simulink model "main_RI_LIEKF_GNSSOutrage"  (R2023a)
settings: Solver=FixedStepAuto  StartTime=0.0  StopTime=220  FixedStep=0.01  RelTol=1e-3
InitFcn:
  | initNavigation0612_AOA;
values from neighbouring files (symbols this model uses):
  CF_enable = 0    [initNavigation.m]
  dt = 0.01    [initNavigation.m]
  dtDelay = -0.03    [initNavigation.m]
  g0 = 9.795    [initNavigation.m]
  gam0_rad = 0/57.3    (= 0)    [initNavigation.m]
  GNSSoutragetime = 90    [initNavigation.m]
  H_sensor_type = 0    [initNavigation.m]
  KF_enable = 1    [initNavigation.m]
  P0 = diag([1*ones(3,1);0.01*ones(3,1);0.1*ones(3,1);0.001*ones(3,1);0.00001*ones(3,1)])    [initNavigation.m]
  P0_RIEKF = diag([1*ones(3,1);0.01*ones(3,1);0.1*ones(3,1);0.001*ones(3,1);0.00001*ones(3,1);      0.01*ones(3,1);[0;2;2]/57.3;[0.1;0.1;0.1]])^2    [initNavigation.m]
  pd0 = 0    [initNavigation.m]
  pe0 = 0    [initNavigation.m]
  phi0_rad = 0/57.3    (= 0)    [initNavigation.m]
  pn0 = 0    [initNavigation.m]
  psi = -178    [initNavigation.m]
  psi0_rad = 0/57.3    (= 0)    [initNavigation.m]
  state_dim = 24    [initNavigation.m]
  Time = 0:0.01:(size(traindata.AttackAngle,1) - 1)*0.01    [NNLiftCoefficientFit.m]
  vd0 = 0    [initNavigation.m]
  ve0 = 0    [initNavigation.m]
  vn0 = 0    [initNavigation.m]
undefined symbols (not defined in the file or in its folder): DiscIntNeverNeededParam, Discrete, INS_CONST, INS_EXPORT, INS_PARAM, magnitude, p, param, pInitialization, sys
libraries: simulink_extras x94, simulink x82, dspstat3 x70, sharedtransform x60, ctrlSharedLib x36, sharedTrackingLibrary x22, matrix_library x15, FMT_Model_Lib x13, deeplib x8, dspsolvers x4, vrlib x4, aerolibconvert2 x1
(part 9 of 28)

== system main_RI_LIEKF_GNSSOutrage/State estimation/bak1/Error State Kalman Filter ==
  Sensor_data : Inport
  INS state : Inport  Port=2
  Add1 : Sum  Inputs=+-
  Add2 : Sum  Inputs=+-
  Bus Creator : BusCreator  Inputs=5
  Bus Selector : BusSelector  OutputSignals=QGC_sensor_reinit,GPS_Data.pos_N_gps,GPS_Data.pos_E_gps,GPS_Data.pos_D_gps,GPS_Data.vn_gps,GPS_Data.ve_gps,GPS_Data.vd_gps
  Bus Selector2 : BusSelector  OutputSignals=RotationData.DCM_b_n,INSstate_v,INSstste_p,INSstate_w,INSstate_fb
  Cal Q1 : Subsystem
  Constant1 : Constant  Value=diag([0.001,0.001,0.001,0.001,0.001,0.001])  OutDataTypeStr=single
  Data Store Read1 : DataStoreRead  DataStoreName=feedback_flag_18dim  IndexOptions=Index vector (dialog)  Indices=1  OutputSizes=1
  Data Store Read2 : DataStoreRead  DataStoreName=GPS_enable  IndexOptions=Index vector (dialog)  Indices=1  OutputSizes=1
  Data Store Read4 : DataStoreRead  DataStoreName=GPS_enable  IndexOptions=Index vector (dialog)  Indices=1  OutputSizes=1
  Data Store Read5 : DataStoreRead  DataStoreName=GPS_enable  IndexOptions=Index vector (dialog)  Indices=1  OutputSizes=1
  Data Store Read6 : DataStoreRead  DataStoreName=feedback_flag_18dim  IndexOptions=Index vector (dialog)  Indices=1  OutputSizes=1
  Data Store Write : DataStoreWrite  DataStoreName=GPS_enable  IndexOptions=Index vector (dialog)  Indices=1  OutputSizes=1
  Data Type Conversion{,1..2,6} (4 alike) : DataTypeConversion  OutDataTypeStr=single  SaturateOnIntegerOverflow=off  RndMeth=Floor
  Extended Kalman Filter1 : Subsystem  mask(Extended Kalman Filter){StateTransitionFcn=stateTransitionFcn_Dyn, HasStateTransitionJacobianFcn=off, StateTransitionJacobianFcn=stateTransitionJacobianFcn_Dyn, HasAdditiveProcessNoise=Nonadditive, ProcessNoise=1, HasTimeVaryingProcessNoise=on, HasStateTransitionFcnExtraArgument=0, InitialState=zeros(15,1), InitialStateCovariance=P0_RIEKF, MeasurementFcn1=GPSMeasurementFcn_Dyn, HasMeasurementJacobianFcn1=off, MeasurementJacobianFcn1=, HasMeasurementEnablePort1=on, HasAdditiveMeasurementNoise1=Nonadditive, MeasurementNoise1=1, HasTimeVaryingMeasurementNoise1=on, HasMeasurementFcnExtraArgument1=0, HasMeasurementWrapping1=off, MeasurementFcn2=ZUPTMeasurementFcn2, HasMeasurementJacobianFcn2=off, MeasurementJacobianFcn2=, HasMeasurementEnablePort2=on, HasAdditiveMeasurementNoise2=Nonadditive, MeasurementNoise2=1, HasTimeVaryingMeasurementNoise2=on, HasMeasurementFcnExtraArgument2=0, HasMeasurementWrapping2=off, MeasurementFcn3=ZUPTMeasurementFcn2, HasMeasurementJacobianFcn3=off, MeasurementJacobianFcn3=, HasMeasurementEnablePort3=on, HasAdditiveMeasurementNoise3=Nonadditive, MeasurementNoise3=1, HasTimeVaryingMeasurementNoise3=on, HasMeasurementFcnExtraArgument3=0, HasMeasurementWrapping3=off, MeasurementFcn4=myMeasurementFcn, HasMeasurementJacobianFcn4=off, MeasurementJacobianFcn4=, HasMeasurementEnablePort4=off, HasAdditiveMeasurementNoise4=Additive, MeasurementNoise4=1, HasTimeVaryingMeasurementNoise4=off, HasMeasurementFcnExtraArgument4=0, HasMeasurementWrapping4=off, MeasurementFcn5=myMeasurementFcn, HasMeasurementJacobianFcn5=off, MeasurementJacobianFcn5=, HasMeasurementEnablePort5=off, HasAdditiveMeasurementNoise5=Additive, MeasurementNoise5=1, HasTimeVaryingMeasurementNoise5=off, HasMeasurementFcnExtraArgument5=0, HasMeasurementWrapping5=off, EnableMultirate=off, StateTransitionFcnSampleTime=0.01, MeasurementFcn1SampleTime=0.2, MeasurementFcn2SampleTime=0.01, MeasurementFcn3SampleTime=1, MeasurementFcn4SampleTime=1, MeasurementFcn5SampleTime=1, UseCurrentEstimator=on, OutputStateCovariance=on, DataType=single, SampleTime=0.01, NumberOfMeasurements=1}
      mask prompts: HasStateTransitionJacobianFcn "shared_tracking:blocks:maskPromptEKFJacobian"; HasTimeVaryingProcessNoise "shared_tracking:blocks:maskPromptEKFUKFTimeVarying"; HasMeasurementJacobianFcn1 "shared_tracking:blocks:maskPromptEKFJacobian"; HasMeasurementEnablePort1 "shared_tracking:blocks:maskPromptEnablePort"; HasTimeVaryingMeasurementNoise1 "shared_tracking:blocks:maskPromptEKFUKFTimeVarying"; HasMeasurementWrapping1 "shared_tracking:blocks:maskPromptEKFUKFMeasurementWrapping"; HasMeasurementJacobianFcn2 "shared_tracking:blocks:maskPromptEKFJacobian"; HasMeasurementEnablePort2 "shared_tracking:blocks:maskPromptEnablePort"; HasTimeVaryingMeasurementNoise2 "shared_tracking:blocks:maskPromptEKFUKFTimeVarying"; HasMeasurementWrapping2 "shared_tracking:blocks:maskPromptEKFUKFMeasurementWrapping"; HasMeasurementJacobianFcn3 "shared_tracking:blocks:maskPromptEKFJacobian"; HasMeasurementEnablePort3 "shared_tracking:blocks:maskPromptEnablePort"; HasTimeVaryingMeasurementNoise3 "shared_tracking:blocks:maskPromptEKFUKFTimeVarying"; HasMeasurementWrapping3 "shared_tracking:blocks:maskPromptEKFUKFMeasurementWrapping"; HasMeasurementJacobianFcn4 "shared_tracking:blocks:maskPromptEKFJacobian"; HasMeasurementEnablePort4 "shared_tracking:blocks:maskPromptEnablePort"; HasTimeVaryingMeasurementNoise4 "shared_tracking:blocks:maskPromptEKFUKFTimeVarying"; HasMeasurementWrapping4 "shared_tracking:blocks:maskPromptEKFUKFMeasurementWrapping"; HasMeasurementJacobianFcn5 "shared_tracking:blocks:maskPromptEKFJacobian"; HasMeasurementEnablePort5 "shared_tracking:blocks:maskPromptEnablePort"; HasTimeVaryingMeasurementNoise5 "shared_tracking:blocks:maskPromptEKFUKFTimeVarying"; HasMeasurementWrapping5 "shared_tracking:blocks:maskPromptEKFUKFMeasurementWrapping"; EnableMultirate "shared_tracking:blocks:maskPromptEnableMultirate"; StateTransitionFcnSampleTime "shared_tracking:blocks:maskPromptStateTransition"; MeasurementFcn1SampleTime "shared_tracking:blocks:maskPromptMeasurement1"; MeasurementFcn2SampleTime "shared_tracking:blocks:maskPromptMeasurement2"; MeasurementFcn3SampleTime "shared_tracking:blocks:maskPromptMeasurement3"; MeasurementFcn4SampleTime "shared_tracking:blocks:maskPromptMeasurement4"; MeasurementFcn5SampleTime "shared_tracking:blocks:maskPromptMeasurement5"; UseCurrentEstimator "shared_tracking:blocks:maskPromptUseCurrentEstimator"; OutputStateCovariance "shared_tracking:blocks:maskPromptOutputStateCovariance"; DataType "shared_tracking:blocks:maskPromptDataType"; SampleTime "shared_tracking:blocks:maskPromptSampleTime"
      mask help: shared_tracking:blocks:maskPromptEKFDescription
      mask init:
      | matlabshared.tracking.internal.blocks.maskInitializationScriptEKF
      mask Help: eval('matlabshared.tracking.internal.blocks.controlIdentLaunchDocPage(''EKF'')')
      mask Callback HasStateTransitionJacobianFcn: matlabshared.tracking.internal.blocks.dialogCallbacksEKFUKFPF(gcbh(),'checkBoxHasJacobianFcn','StateTransition');
      mask TypeOptions HasAdditiveProcessNoise: shared_tracking:blocks:maskPromptEKFUKFAdditiveNoise | shared_tracking:blocks:maskPromptEKFUKFNonAdditiveNoise
      mask Callback HasTimeVaryingProcessNoise: matlabshared.tracking.internal.blocks.dialogCallbacksEKFUKFPF(gcbh,'checkboxIsCovarianceTimeVarying','HasTimeVaryingProcessNoise','ProcessNoise')
      mask Callback HasMeasurementJacobianFcn1: matlabshared.tracking.internal.blocks.dialogCallbacksEKFUKFPF(gcbh(),'checkBoxHasJacobianFcn','Measurement','1');
      mask TypeOptions HasAdditiveMeasurementNoise1: shared_tracking:blocks:maskPromptEKFUKFAdditiveNoise | shared_tracking:blocks:maskPromptEKFUKFNonAdditiveNoise
      mask Callback HasTimeVaryingMeasurementNoise1: matlabshared.tracking.internal.blocks.dialogCallbacksEKFUKFPF(gcbh,'checkboxIsCovarianceTimeVarying','HasTimeVaryingMeasurementNoise1','MeasurementNoise1')
      mask Callback HasMeasurementJacobianFcn2: matlabshared.tracking.internal.blocks.dialogCallbacksEKFUKFPF(gcbh(),'checkBoxHasJacobianFcn','Measurement','2');
      mask TypeOptions HasAdditiveMeasurementNoise2: shared_tracking:blocks:maskPromptEKFUKFAdditiveNoise | shared_tracking:blocks:maskPromptEKFUKFNonAdditiveNoise
      mask Callback HasTimeVaryingMeasurementNoise2: matlabshared.tracking.internal.blocks.dialogCallbacksEKFUKFPF(gcbh,'checkboxIsCovarianceTimeVarying','HasTimeVaryingMeasurementNoise2','MeasurementNoise2')
      mask Callback HasMeasurementJacobianFcn3: matlabshared.tracking.internal.blocks.dialogCallbacksEKFUKFPF(gcbh(),'checkBoxHasJacobianFcn','Measurement','3');
      mask TypeOptions HasAdditiveMeasurementNoise3: shared_tracking:blocks:maskPromptEKFUKFAdditiveNoise | shared_tracking:blocks:maskPromptEKFUKFNonAdditiveNoise
      mask Callback HasTimeVaryingMeasurementNoise3: matlabshared.tracking.internal.blocks.dialogCallbacksEKFUKFPF(gcbh,'checkboxIsCovarianceTimeVarying','HasTimeVaryingMeasurementNoise3','MeasurementNoise3')
      mask Callback HasMeasurementJacobianFcn4: matlabshared.tracking.internal.blocks.dialogCallbacksEKFUKFPF(gcbh(),'checkBoxHasJacobianFcn','Measurement','4');
      mask TypeOptions HasAdditiveMeasurementNoise4: shared_tracking:blocks:maskPromptEKFUKFAdditiveNoise | shared_tracking:blocks:maskPromptEKFUKFNonAdditiveNoise
      mask Callback HasTimeVaryingMeasurementNoise4: matlabshared.tracking.internal.blocks.dialogCallbacksEKFUKFPF(gcbh,'checkboxIsCovarianceTimeVarying','HasTimeVaryingMeasurementNoise4','MeasurementNoise4')
      mask Callback HasMeasurementJacobianFcn5: matlabshared.tracking.internal.blocks.dialogCallbacksEKFUKFPF(gcbh(),'checkBoxHasJacobianFcn','Measurement','5');
      mask TypeOptions HasAdditiveMeasurementNoise5: shared_tracking:blocks:maskPromptEKFUKFAdditiveNoise | shared_tracking:blocks:maskPromptEKFUKFNonAdditiveNoise
      mask Callback HasTimeVaryingMeasurementNoise5: matlabshared.tracking.internal.blocks.dialogCallbacksEKFUKFPF(gcbh,'checkboxIsCovarianceTimeVarying','HasTimeVaryingMeasurementNoise5','MeasurementNoise5')
      mask Callback EnableMultirate: matlabshared.tracking.internal.blocks.dialogCallbacksEKFUKFPF(gcbh,'checkBoxHasMultirate')
      mask TypeOptions DataType: shared_tracking:blocks:maskPromptDouble | shared_tracking:blocks:maskPromptSingle
      mask Callback NumberOfMeasurements: matlabshared.tracking.internal.blocks.dialogCallbacksEKFUKFPF(gcbh,'editboxNumberOfMeasurements','MeasurementFcn');
      mask DialogControl DescGroupVar Prompt: shared_tracking:blocks:maskPromptEKFTitle
      mask DialogControl TabSystemModel Prompt: shared_tracking:blocks:maskPromptSystemModel
      mask DialogControl GroupStateTransition Prompt: shared_tracking:blocks:maskPromptStateTransition
      mask DialogControl StateTransitionFunctionText Prompt: shared_tracking:blocks:maskPromptFunction
      mask DialogControl HasStateTransitionJacobianFcn Prompt: Jacobian
      mask DialogControl ProcessNoiseText Prompt: shared_tracking:blocks:maskPromptEKFUKFProcessNoise
      mask DialogControl ProcessNoiseCovarianceText Prompt: shared_tracking:blocks:maskPromptCovariance
      mask DialogControl HasTimeVaryingProcessNoise Prompt: Time-varying
      mask DialogControl InitializationContainer Prompt: shared_tracking:blocks:maskPromptInitialization
      mask DialogControl InitialStateText Prompt: shared_tracking:blocks:maskPromptEKFUKFInitialState
      mask DialogControl InitialCovarianceText Prompt: shared_tracking:blocks:maskPromptEKFUKFInitialCovariance
      mask DialogControl GroupMeasurement1 Prompt: shared_tracking:blocks:maskPromptMeasurement1
      mask DialogControl MeasurementFunction1Text Prompt: shared_tracking:blocks:maskPromptFunction
      mask DialogControl HasMeasurementJacobianFcn1 Prompt: Jacobian
      mask DialogControl HasMeasurementEnablePort1 Prompt: Add Enable port
      mask DialogControl MeasurementNoiseText1 Prompt: shared_tracking:blocks:maskPromptEKFUKFMeasurementNoise
      mask DialogControl MeasurementNoiseCovarianceText1 Prompt: shared_tracking:blocks:maskPromptCovariance
      mask DialogControl HasTimeVaryingMeasurementNoise1 Prompt: Time-varying
      mask DialogControl HasMeasurementWrapping1 Prompt: Has measurement wrapping
      mask DialogControl GroupMeasurement2 Prompt: shared_tracking:blocks:maskPromptMeasurement2
      mask DialogControl MeasurementFunction2Text Prompt: shared_tracking:blocks:maskPromptFunction
      mask DialogControl HasMeasurementJacobianFcn2 Prompt: Jacobian
      mask DialogControl HasMeasurementEnablePort2 Prompt: Add Enable port
      mask DialogControl MeasurementNoiseText2 Prompt: shared_tracking:blocks:maskPromptEKFUKFMeasurementNoise
      mask DialogControl MeasurementNoiseCovarianceText2 Prompt: shared_tracking:blocks:maskPromptCovariance
      mask DialogControl HasTimeVaryingMeasurementNoise2 Prompt: Time-varying
      mask DialogControl HasMeasurementWrapping2 Prompt: Has measurement wrapping
      mask DialogControl GroupMeasurement3 Prompt: shared_tracking:blocks:maskPromptMeasurement3
      mask DialogControl MeasurementFunction3Text Prompt: shared_tracking:blocks:maskPromptFunction
      mask DialogControl HasMeasurementJacobianFcn3 Prompt: Jacobian
      mask DialogControl HasMeasurementEnablePort3 Prompt: Add Enable port
      mask DialogControl MeasurementNoiseText3 Prompt: shared_tracking:blocks:maskPromptEKFUKFMeasurementNoise
      mask DialogControl MeasurementNoiseCovarianceText3 Prompt: shared_tracking:blocks:maskPromptCovariance
      mask DialogControl HasTimeVaryingMeasurementNoise3 Prompt: Time-varying
      mask DialogControl HasMeasurementWrapping3 Prompt: Has measurement wrapping
      mask DialogControl GroupMeasurement4 Prompt: shared_tracking:blocks:maskPromptMeasurement4
      mask DialogControl MeasurementFunction4Text Prompt: shared_tracking:blocks:maskPromptFunction
      mask DialogControl HasMeasurementJacobianFcn4 Prompt: Jacobian
      mask DialogControl HasMeasurementEnablePort4 Prompt: Add Enable port
      mask DialogControl MeasurementNoiseText4 Prompt: shared_tracking:blocks:maskPromptEKFUKFMeasurementNoise
      mask DialogControl MeasurementNoiseCovarianceText4 Prompt: shared_tracking:blocks:maskPromptCovariance
      mask DialogControl HasTimeVaryingMeasurementNoise4 Prompt: Time-varying
      mask DialogControl HasMeasurementWrapping4 Prompt: Has measurement wrapping
      mask DialogControl GroupMeasurement5 Prompt: shared_tracking:blocks:maskPromptMeasurement5
      mask DialogControl MeasurementFunction5Text Prompt: shared_tracking:blocks:maskPromptFunction
      mask DialogControl HasMeasurementJacobianFcn5 Prompt: Jacobian
      mask DialogControl HasMeasurementEnablePort5 Prompt: Add Enable port
      mask DialogControl MeasurementNoiseText5 Prompt: shared_tracking:blocks:maskPromptEKFUKFMeasurementNoise
      mask DialogControl MeasurementNoiseCovarianceText5 Prompt: shared_tracking:blocks:maskPromptCovariance
      mask DialogControl HasTimeVaryingMeasurementNoise5 Prompt: Time-varying
      mask DialogControl HasMeasurementWrapping5 Prompt: Has measurement wrapping
      mask DialogControl AddMeasurement Prompt: shared_tracking:blocks:maskPromptAddMeasurement
      mask DialogControl AddMeasurement Callback: matlabshared.tracking.internal.blocks.dialogCallbacksEKFUKFPF(gcbh,'buttonAddMeasurement','MeasurementFcn');
      mask DialogControl RemoveMeasurement Prompt: shared_tracking:blocks:maskPromptRemoveMeasurement
      mask DialogControl RemoveMeasurement Callback: matlabshared.tracking.internal.blocks.dialogCallbacksEKFUKFPF(gcbh,'buttonRemoveMeasurement','MeasurementFcn');
      mask DialogControl TabMultirate Prompt: shared_tracking:blocks:maskPromptEKFUKFMultirate
      mask DialogControl GroupMultirate Prompt: shared_tracking:blocks:maskPromptEKFUKFMultirate
      mask DialogControl EnableMultirate Prompt: Enable multirate operation
      mask DialogControl GroupMultirateSampleTimes Prompt: shared_tracking:blocks:maskPromptSampleTimeNoInheritance
      mask DialogControl StateTransitionFcnSampleTime Prompt: State Transition
      mask DialogControl MeasurementFcn1SampleTime Prompt: Measurement 1
      mask DialogControl MeasurementFcn2SampleTime Prompt: Measurement 2
      mask DialogControl MeasurementFcn3SampleTime Prompt: Measurement 3
      mask DialogControl MeasurementFcn4SampleTime Prompt: Measurement 4
      mask DialogControl MeasurementFcn5SampleTime Prompt: Measurement 5
      mask DialogControl ContainerSettings Prompt: shared_tracking:blocks:maskPromptEKFUKFSettings
      mask DialogControl UseCurrentEstimator Prompt: Use the current measurements to improve state estimates
      mask DialogControl OutputStateCovariance Prompt: Output state estimation error covariance
      mask DialogControl DataType Prompt: Data type:
      mask DialogControl SampleTime Prompt: Sample time:
  Extract Diagonal1 : matrix_library/Extract Diagonal
  From1 : From  Commented=on  GotoTag=wxyz
  From11 : From  Commented=on  GotoTag=wxyz
  From13 : From  Commented=on  GotoTag=fbxyz
  From14 : From  Commented=on  GotoTag=DCM_b_n
  From2 : From  Commented=on  GotoTag=fbxyz
  From3 : From  Commented=on  GotoTag=ZUPTenable
  From5 : From  Commented=on  GotoTag=fex
  From6 : From  Commented=on  GotoTag=DCM_b_n
  From9 : From  Commented=on  GotoTag=DCM_b_n
  Goto6 : Goto  Commented=on  GotoTag=ZUPTenable
  MATLAB Function : MATLAB Function  TreatAsAtomicUnit=on
  MATLAB Function1 : MATLAB Function  Commented=on  TreatAsAtomicUnit=on
  Memory : Memory
  Memory1 : Memory  Commented=on
  Mux : Mux  Inputs=3
  Mux1 : Mux  Inputs=3
  Mux2 : Mux  Inputs=2
  RIEKF : MATLAB Function  Commented=on  TreatAsAtomicUnit=on
  Rate Transition2 : RateTransition  Commented=on  OutPortSampleTime=dt
  Rate Transition{5..8} (4 alike) : RateTransition  OutPortSampleTime=dt
  Scope{,1,5..7} (5 alike) : Scope
  Scope10 : Scope  Commented=on  NumInputPorts=2
  Scope8 : Scope  NumInputPorts=2
  Simulink Function - GPS Measurements : Subsystem  TreatAsAtomicUnit=on
  Simulink Function - GPS Measurements1 : Subsystem  Commented=on  TreatAsAtomicUnit=on
  Simulink Function - GPS Measurements2 : Subsystem  Commented=on  TreatAsAtomicUnit=on
  Simulink Function - State Transition : Subsystem  TreatAsAtomicUnit=on
  Simulink Function - State Transition Jacobian : Subsystem  Commented=on  TreatAsAtomicUnit=on
  Subsystem : Subsystem
  Unscented Kalman Filter1 : sharedTrackingLibrary/Unscented Kalman Filter  Commented=on  StateTransitionFcn=stateTransitionFcn_Dyn  HasAdditiveProcessNoise=Nonadditive  ProcessNoise=1  HasTimeVaryingProcessNoise=on  HasStateTransitionFcnExtraArgument=0  InitialState=zeros(18,1)  InitialStateCovariance=diag([1*ones(3,1);0.1*ones(3,1);0.001*ones(3,1);0.001*ones(6,1);0.1*ones(3,1)]);  Alpha=1e-2  Beta=2  Kappa=0  MeasurementFcn1=GPSMeasurementFcn_Dyn  HasMeasurementEnablePort1=on  HasAdditiveMeasurementNoise1=Nonadditive  MeasurementNoise1=1  HasTimeVaryingMeasurementNoise1=on  HasMeasurementFcnExtraArgument1=0  HasMeasurementWrapping1=off  MeasurementFcn2=DynamicMeasurementFcn_Dyn  HasMeasurementEnablePort2=on  HasAdditiveMeasurementNoise2=Nonadditive  MeasurementNoise2=1  HasTimeVaryingMeasurementNoise2=on  HasMeasurementFcnExtraArgument2=0  HasMeasurementWrapping2=off  MeasurementFcn3=myMeasurementFcn  HasMeasurementEnablePort3=off  HasAdditiveMeasurementNoise3=Additive  MeasurementNoise3=1  HasTimeVaryingMeasurementNoise3=off  HasMeasurementFcnExtraArgument3=0  HasMeasurementWrapping3=off  MeasurementFcn4=myMeasurementFcn  HasMeasurementEnablePort4=off  HasAdditiveMeasurementNoise4=Additive  MeasurementNoise4=1  HasTimeVaryingMeasurementNoise4=off  HasMeasurementFcnExtraArgument4=0  HasMeasurementWrapping4=off  MeasurementFcn5=myMeasurementFcn  HasMeasurementEnablePort5=off  HasAdditiveMeasurementNoise5=Additive  MeasurementNoise5=1  HasTimeVaryingMeasurementNoise5=off  HasMeasurementFcnExtraArgument5=0  HasMeasurementWrapping5=off  EnableMultirate=off  StateTransitionFcnSampleTime=1  MeasurementFcn1SampleTime=1  MeasurementFcn2SampleTime=1  MeasurementFcn3SampleTime=1  MeasurementFcn4SampleTime=1  MeasurementFcn5SampleTime=1  UseCurrentEstimator=on  OutputStateCovariance=on  DataType=single  SampleTime=0.01  NumberOfMeasurements=2
  delta_state : Outport
  Measuemrnt Enable Flag : Outport  Port=2
  covariance : Outport  Port=3
  wires:
  Add1/1 -> Data Type Conversion/1
  Add2/1 -> Data Type Conversion2/1
  [p_INS] -> Add1/1
  [v_INS] -> Add2/1
  Mux2/1 -> Rate Transition7/1, Scope1/1
  Data Type Conversion2/1 -> Mux2/1
  Data Type Conversion/1 -> Mux2/2
  [pos_NED] -> Add1/2
  [vel_NED] -> Add2/2
  [DCM_b_n] -> Simulink Function - GPS Measurements/1(Rbn)
  [p_INS] -> Simulink Function - GPS Measurements/3(pn)
  [v_INS] -> Simulink Function - GPS Measurements/2(vn)
  [p_INS] -> Simulink Function - State Transition/3(pn)
  [v_INS] -> Simulink Function - State Transition/2(vn)
  Rate Transition2/1 -> ?
  From3/1 -> Rate Transition2/1
  Data Store Read4/1 -> Measuemrnt Enable Flag/1
  Data Store Read2/1 -> Rate Transition6/1
  From6/1 -> MATLAB Function1/1(Cbn)
  MATLAB Function1/2(ZeroVelDetectFlagold) -> Scope10/2
  Memory1/1 -> MATLAB Function1/4(fex)
  From5/1 -> Memory1/1
  Mux/1 -> [pos_NED]
  From1/1 -> MATLAB Function1/2(wxyz)
  MATLAB Function1/1(ZeroVelDetectFlag) -> Goto6/1, Scope10/1
  From2/1 -> MATLAB Function1/3(fbxyz)
  Bus Selector2/2 -> [v_INS]  "<INSstate_v>"
  Data Store Read6/1 -> Scope8/2
  Data Store Read5/1 -> Scope8/1
  Data Type Conversion6/1 -> Extended Kalman Filter1/1(Q)
  Rate Transition5/1 -> Data Type Conversion6/1
  Cal Q1/1(Qd) -> Rate Transition5/1
  Rate Transition8/1 -> Extended Kalman Filter1/4(R1)
  Rate Transition7/1 -> Extended Kalman Filter1/3(y1)
  Rate Transition6/1 -> Extended Kalman Filter1/2(Enable1)
  Extract Diagonal1/1 -> Scope6/1, covariance/1
  Extended Kalman Filter1/2(P) -> Extract Diagonal1/1
  Constant1/1 -> Rate Transition8/1
  From14/1 -> Simulink Function - GPS Measurements1/1(DCM_b_n)
  From13/1 -> Simulink Function - State Transition Jacobian/3(fbxyz)
  From11/1 -> Simulink Function - State Transition Jacobian/2(wxyz)
  From9/1 -> Simulink Function - State Transition Jacobian/1(DCM_b_n)
  [DCM_b_n] -> Simulink Function - State Transition/1(DCM_b_n)
  MATLAB Function/3(dtheta) -> Bus Creator/3  "KFState_dtheta"
  MATLAB Function/1(dp) -> Bus Creator/1  "KFState_dp"
  Extended Kalman Filter1/1(xhat) -> Data Type Conversion1/1, Scope/1
  Subsystem/1(flag) -> Scope5/1, Data Store Write/1
  [pos_NED] -> Subsystem/1(data)
  Data Store Read1/1 -> Scope7/1
  Bus Selector/6 -> Mux1/2  "<ve_gps>"
  Sensor_data/1 -> Bus Selector/1
  Mux1/1 -> [vel_NED]
  Bus Selector/5 -> Mux1/1  "<vn_gps>"
  Bus Selector/7 -> Mux1/3  "<vd_gps>"
  Bus Selector/3 -> Mux/2  "<pos_E_gps>"
  Bus Selector/2 -> Mux/1  "<pos_N_gps>"
  Bus Selector/4 -> Mux/3  "<pos_D_gps>"
  INS state/1 -> Bus Selector2/1
  Bus Selector2/4 -> [wxyz]  "<INSstate_w>"
  Bus Selector2/5 -> [fbxyz]  "<INSstate_fb>"
  Bus Selector2/1 -> [DCM_b_n]  "<DCM_b_n>"
  Bus Selector2/3 -> [p_INS]  "<INSstste_p>"
  MATLAB Function/4(da) -> Bus Creator/4  "KFState_da"
  MATLAB Function/2(dv) -> Bus Creator/2  "KFState_dv"
  MATLAB Function/5(dg) -> Bus Creator/5  "KFState_dg"
  Data Type Conversion1/1 -> Memory/1
  Bus Creator/1 -> delta_state/1
  Memory/1 -> MATLAB Function/1(u)

== system main_RI_LIEKF_GNSSOutrage/State estimation/bak1/INS propogation ==
  note: q(1:3)
  Sensor_data : Inport
  Measuemrnt Enable Flag : Inport  Port=2
  delta_state : Inport  Port=3
  Bus Creator : BusCreator  Inputs=7
  Bus Selector : BusSelector  OutputSignals=IMU_Data.gyro_B_rad/s_LPF,IMU_Data.accl_B_m/s2_LPF,MAGN_Data,QGC_sensor_reinit,GPS_Data.pos_N_gps,GPS_Data.pos_E_gps,GPS_Data.pos_D_gps,GPS_Data.vn_gps,GPS_Data.ve_gps,GPS_Data.vd_gps
  Bus Selector1 : BusSelector  OutputSignals=DCM_b_n
  Bus Selector2 : BusSelector  OutputSignals=KFState_dp,KFState_dv,KFState_dtheta,KFState_da,KFState_dg
  Data Type Conversion : DataTypeConversion  OutDataTypeStr=single  SaturateOnIntegerOverflow=off  RndMeth=Floor
  Init_PVQ : Subsystem
  Mux : Mux  Inputs=3
  Mux1 : Mux  Inputs=3
  Scope1 : Scope
  accl bias compensation : Subsystem
  att_update : Subsystem
  gyro bias compensation : Subsystem
  vel_pos_update : Subsystem
  INSstate : Outport
  wires:
  [dda] -> ?
  [ddg] -> ?
  [dtheta] -> vel_pos_update/1(dtheta)
  Mux/1 -> [pos_NED]
  Init_PVQ/1(quat_0) -> att_update/3(quat_0)
  [fbxyz] -> vel_pos_update/3(Ab)
  [QGC_init] -> att_update/4(init_flag)
  Bus Selector/10 -> Mux1/3  "<vd_gps>"
  [vel_NED] -> Data Type Conversion/1
  Bus Selector/7 -> Mux/3  "<pos_D_gps>"
  Bus Selector/8 -> Mux1/1  "<vn_gps>"
  Bus Selector/5 -> Mux/1  "<pos_N_gps>"
  [dtheta] -> att_update/1(dtheta)
  [wxyz] -> att_update/2(gyro)
  Bus Selector/6 -> Mux/2  "<pos_E_gps>"
  Bus Selector/3 -> [Magn]  "<MAGN_Data>"
  Mux1/1 -> [vel_NED]
  Sensor_data/1 -> Bus Selector/1
  [fbxyz] -> Init_PVQ/2(accl_B_m/s2_LPF)
  Init_PVQ/2(v0) -> vel_pos_update/4(v0)
  Init_PVQ/3(p0) -> vel_pos_update/5(p0)
  Bus Selector/9 -> Mux1/2  "<ve_gps>"
  [QGC_init] -> vel_pos_update/6(QGC_init)
  [pos_NED] -> Init_PVQ/4(pos_NED)
  Data Type Conversion/1 -> Init_PVQ/5(vel_NED)
  [dp] -> vel_pos_update/7(dp)
  [Magn] -> Init_PVQ/3(Magn_B_guess_LPF)
  Bus Selector/4 -> [QGC_init]  "<QGC_sensor_reinit>"
  Bus Selector/1 -> [gyro_raw]  "<gyro_B_rad/s_LPF>"
  Bus Selector1/1 -> vel_pos_update/2(<DCM_b_n>), [Cbn]  "<DCM_b_n>"
  vel_pos_update/2(V) -> Bus Creator/3  "INSstate_v"
  [dv] -> vel_pos_update/8(dv)
  [QGC_init] -> Init_PVQ/1(QGC_sensor_reinit)
  vel_pos_update/1(p_k) -> Bus Creator/2  "INSstste_p"
  [wxyz] -> Bus Creator/4  "INSstate_w"
  [fbxyz] -> Bus Creator/5  "INSstate_fb"
  att_update/1(att_update1) -> Bus Creator/1, Bus Selector1/1  "RotationData"
  Bus Creator/1 -> INSstate/1
  accl bias compensation/1(fb) -> [fbxyz]
  accl bias compensation/2(da) -> [da]
  Measuemrnt Enable Flag/1 -> gyro bias compensation/3(Measuemrnt Enable Flag)
  gyro bias compensation/1(wb) -> [wxyz]
  gyro bias compensation/2(dg) -> [dg]
  [dg] -> Bus Creator/6  "INSstate_dg"
  [da] -> Bus Creator/7  "INSstate_da"
  delta_state/1 -> Bus Selector2/1, Scope1/1
  Bus Selector2/1 -> [dp]  "<KFState_dp>"
  Bus Selector2/2 -> [dv]  "<KFState_dv>"
  Bus Selector2/3 -> [dtheta]  "<KFState_dtheta>"
  Bus Selector2/4 -> [dda]  "<KFState_da>"
  Bus Selector2/5 -> [ddg]  "<KFState_dg>"
  [gyro_raw] -> gyro bias compensation/1(raw <gyro_B_rad/s_LPF>)
  [accl_raw] -> accl bias compensation/1(raw <accl_B_m/s2_LPF>)
  Bus Selector/2 -> [accl_raw]  "<accl_B_m/s2_LPF>"

== system main_RI_LIEKF_GNSSOutrage/State estimation/distribute CF/AHRS ==
  <QGC_sensor_reinit> : Inport  PortDimensions=1
  <accl_B_m/s2_LPF> : Inport  Port=2  PortDimensions=3
  <MAGN_Data> : Inport  Port=3  PortDimensions=3
  <GPS_Data> : Inport  Port=4
  Sensor_data : Inport  Port=5
  <QGC_sensor_reinit>1 : InportShadow  PortDimensions=1
  <QGC_sensor_reinit>2 : InportShadow  PortDimensions=1
  AHRS Complementary filter : Subsystem  mask{GPS_accel_kp=0.3, GPS_accel_ki=0.05, noGPS_accel_kp=0.3, noGPS_accel_ki=0.05}
      mask prompts: GPS_accel_kp "GPS修正下互补滤波增益kp"; GPS_accel_ki "GPS修正下互补滤波增益Ki"; noGPS_accel_kp "无GPS修正下互补滤波增益kp"; noGPS_accel_ki "无GPS修正下互补滤波增益Ki"
      mask DialogControl DescTextVar Prompt: AHRS Complementary filter
  Bus Selector1 : BusSelector  OutputSignals=IMU_Data.accl_B_m/s2_LPF
  Bus Selector2 : BusSelector  OutputSignals=MAGN_Data
  Init_Q0 : Subsystem
  Scope : Scope
  Scope1 : Scope
  Sensor_data_1 : InportShadow  Port=5
  att_update : Subsystem
  RotationData : Outport
  wires:
  <QGC_sensor_reinit>2/1 -> AHRS Complementary filter/5(reset)
  <GPS_Data>/1 -> AHRS Complementary filter/3(GPS_Data)
  att_update/1(att_update) -> RotationData/1, AHRS Complementary filter/2(Q_update)
  Init_Q0/1(quat_0) -> att_update/2(quat_0), Scope1/1
  <MAGN_Data>/1 -> Init_Q0/3(Magn_B_guess_LPF)
  <accl_B_m/s2_LPF>/1 -> Init_Q0/2(accl_B_m/s2_LPF)
  <QGC_sensor_reinit>/1 -> Init_Q0/1(QGC_sensor_reinit)
  AHRS Complementary filter/1(w_bias) -> Scope/1, att_update/4(wbias)
  <QGC_sensor_reinit>1/1 -> att_update/3(init_flag)
  Bus Selector2/1 -> AHRS Complementary filter/4(magxyz)  "<MAGN_Data>"
  Bus Selector1/1 -> AHRS Complementary filter/1(fbxyz)  "<accl_B_m/s2_LPF>"
  Sensor_data_1/1 -> Bus Selector1/1, Bus Selector2/1
  Sensor_data/1 -> att_update/1(Sensor_data)

== system main_RI_LIEKF_GNSSOutrage/State estimation/distribute CF/Translation_estimate ==
  RotationData : Inport
  Sensor_data : Inport  Port=2
  Add : Sum  Inputs=++-
  Bus Creator2 : BusCreator  Inputs=6
  Bus Selector : BusSelector  OutputSignals=TOF_Data.H_TOF_TD,GPS_Data.pos_D_gps,QGC_sensor_reinit,GPS_Data.fixtype_gps
  Compare To Constant : simulink/Logic and Bit Operations/Compare To Constant  relop=>=  const=1  OutDataTypeStr=boolean
  Constant : Constant
  Constant1 : Constant  Value=H_sensor_type  OutDataTypeStr=single
  Constant2 : Constant  Value=g0  OutDataTypeStr=single
  Demux : Demux  Outputs=2
  Demux1 : Demux  Outputs=2
  Demux2 : Demux  Outputs=3
  Detect Increase : simulink/Logic and Bit Operations/Detect Increase  vinit=0.0  OutDataTypeStr=boolean
  Gain2 : Gain  Gain=-1
  KalmanFilter_altitude : ctrlSharedLib/Kalman Filter  TimeDomain=Discrete-Time  UseCurrentEstimator=on  ModelSource=Individual A, B, C, D matrices  ModelSourceVariable=sys  A=[1 0.01 0; 0 1 -0.01;0 0 1-1/50;]  B=[0;0.01;0]  C=[1 0 0]  D=[0]  NumberOfStates=2  NumberOfInputs=2  NumberOfOutputs=2  InitialEstimateSource=Dialog  X0=[0 0 0]  P0=10  UseK=off  UseGH=on  NumberOfProcessNoiseInputs=2  G=diag([0;1;1])  TimeInvariantG=on  H=0  TimeInvariantH=on  Q=diag([0;5e-3;5e-4])  TimeInvariantQ=on  R=0.1  TimeInvariantR=on  N=0  TimeInvariantN=on  AddInputPort=on  AddEnablePort=on  ExternalReset=Rising  OutputEstimatedY=off  OutputP=off  Ts=-1
  Memory : Memory
  Rxy_Horizontal_estimation : Subsystem
  Scope : Scope  NumInputPorts=2
  Scope2 : Scope
  Sensor_data1 : InportShadow  Port=2
  Switch : Switch  Threshold=1  SaturateOnIntegerOverflow=off  InputSameDT=off
  V_Horizontal_estimation : Subsystem
  Zero-Order Hold : ZeroOrderHold  SampleTime=0.01
  Zero-Order Hold1 : ZeroOrderHold  SampleTime=0.01
  Zero-Order Hold2 : ZeroOrderHold  SampleTime=0.01
  translate to N : Subsystem
  TranslationData : Outport
  wires:
  RotationData/1 -> translate to N/1(RotationData)
  Bus Creator2/1 -> TranslationData/1
  Demux1/2 -> Bus Creator2/5  "pe_m"
  Demux1/1 -> Bus Creator2/4  "pn_m"
  Demux/2 -> Bus Creator2/2  "ve_m/s"
  Demux/1 -> Bus Creator2/1  "vn_m/s"
  translate to N/2(accel_Vertical_predict) -> [accel_Vertical_predict]
  V_Horizontal_estimation/3(GPS_v_enable) -> Rxy_Horizontal_estimation/2(Enable)
  V_Horizontal_estimation/2(V_n&e) -> Rxy_Horizontal_estimation/1(Vn)
  V_Horizontal_estimation/1(vxy_estimout) -> Demux/1  "v_ne_"
  translate to N/1(accel_Horizontal_predict) -> V_Horizontal_estimation/1(An)
  Rxy_Horizontal_estimation/1(R_n&e) -> Demux1/1
  Sensor_data/1 -> translate to N/2(Sensor_data), V_Horizontal_estimation/2(Sensor_data2), Rxy_Horizontal_estimation/3(Sensor_data2)
  Sensor_data1/1 -> Bus Selector/1
  KalmanFilter_altitude/1 -> Demux2/1
  Zero-Order Hold/1 -> KalmanFilter_altitude/1
  Switch/1 -> Zero-Order Hold1/1
  Zero-Order Hold1/1 -> KalmanFilter_altitude/2
  Demux2/2 -> Bus Creator2/3  "vd_m/s"
  Demux2/1 -> Bus Creator2/6  "pd_m"
  [accel_Vertical_predict] -> Scope/1, Add/1
  Add/1 -> Zero-Order Hold/1
  Demux2/3 -> Memory/1
  Memory/1 -> Add/3, Scope/2
  Constant2/1 -> Add/2
  Constant1/1 -> Switch/2
  Bus Selector/1 -> Gain2/1  "<H_TOF_TD>"
  Gain2/1 -> Switch/1
  Bus Selector/3 -> Scope2/1, Detect Increase/1  "<QGC_sensor_reinit>"
  Detect Increase/1 -> KalmanFilter_altitude/4
  Bus Selector/4 -> Zero-Order Hold2/1  "<fixtype_gps>"
  Compare To Constant/1 -> KalmanFilter_altitude/3
  Zero-Order Hold2/1 -> Compare To Constant/1
  Bus Selector/2 -> Switch/3  "<pos_D_gps>"

== system main_RI_LIEKF_GNSSOutrage/State estimation/distribute CF/distribute CF ==
  Sensor_data : Inport
  AHRS1 : Subsystem  Commented=on  TreatAsAtomicUnit=on
  Bus_Constructor : Subsystem  TreatAsAtomicUnit=on
  Correct : Subsystem
  Delay : Delay  DelayLength=1
  Translation_estimate : Subsystem
  Update : Subsystem  TreatAsAtomicUnit=on
  初始化 : Subsystem
  RotationData : Outport
  TranslationData : Outport  Port=2
  wires:
  Sensor_data/1 -> Translation_estimate/2(Sensor_data), Bus_Constructor/6(Sensor_Data), Update/4(Sensor_Data), Correct/1(Sensor_Data), 初始化/1(Sensor_Data)
  Correct/1(att_B_correction) -> Update/1(att_B_correction)
  Correct/2(bias_g_B_correction) -> Update/2(bias_g_correction)
  初始化/1(RF_data) -> Update/3(RF_Data), Bus_Constructor/1(RF_Data)
  Update/1(att_quat) -> Bus_Constructor/2(att_quat)
  Update/2(DCM_OB) -> Bus_Constructor/3(DCM_OB)
  Update/3(bias_g) -> Bus_Constructor/4(bias_g)
  Bus_Constructor/1(Rotation_Data) -> Delay/1, Translation_estimate/1(RotationData), RotationData/1
  Delay/1 -> Correct/2(Rotation_Data)
  Translation_estimate/1(TranslationData) -> TranslationData/1
  Update/4(gyro_B_correction) -> Bus_Constructor/5(gyro_B_correction)

== system main_RI_LIEKF_GNSSOutrage/Sensor_Data_Process/IMU_Data_Process/Bias Eliminate/Subsystem ==
  data : Inport
  Buffer : Buffer  N=50  V=49  OutputFrames=off
  Buffer1 : Buffer  N=50  V=49  OutputFrames=off
  Buffer2 : Buffer  N=50  V=49  OutputFrames=off
  Demux : Demux  Outputs=3
  Mean4 : dspstat3/Mean  run=off  reset_popup=None  directionMode=Entire input  dimension=3  roiEnable=off  roiType=Rectangles  roiPortion=Entire ROI  roiOutput=Individual statistics for each ROI  roiFlag=off  roundingMode=Floor  overflowMode=off  outputDataTypeStr=Inherit: Same as accumulator  outputMin=[]  outputMax=[]  outputLastDataTypeStr=Inherit: Same as accumulator
  Mean5 : dspstat3/Mean  run=off  reset_popup=None  directionMode=Entire input  dimension=3  roiEnable=off  roiType=Rectangles  roiPortion=Entire ROI  roiOutput=Individual statistics for each ROI  roiFlag=off  roundingMode=Floor  overflowMode=off  outputDataTypeStr=Inherit: Same as accumulator  outputMin=[]  outputMax=[]  outputLastDataTypeStr=Inherit: Same as accumulator
  Mean6 : dspstat3/Mean  run=off  reset_popup=None  directionMode=Entire input  dimension=3  roiEnable=off  roiType=Rectangles  roiPortion=Entire ROI  roiOutput=Individual statistics for each ROI  roiFlag=off  roundingMode=Floor  overflowMode=off  outputDataTypeStr=Inherit: Same as accumulator  outputMin=[]  outputMax=[]  outputLastDataTypeStr=Inherit: Same as accumulator
  Scope : Scope  NumInputPorts=2
  Vector Concatenate : Concatenate  NumInputs=3
  mean_data : Outport
  wires:
  data/1 -> Demux/1, Scope/1
  Vector Concatenate/1 -> mean_data/1, Scope/2
  Mean4/1 -> Vector Concatenate/1
  Demux/3 -> Buffer2/1
  Buffer1/1 -> Mean5/1  "fby_buff"
  Demux/1 -> Buffer/1
  Buffer2/1 -> Mean6/1  "fbz_buff"
  Mean5/1 -> Vector Concatenate/2
  Buffer/1 -> Mean4/1  "fbx_buff"
  Demux/2 -> Buffer1/1
  Mean6/1 -> Vector Concatenate/3

== system main_RI_LIEKF_GNSSOutrage/Sensor_Data_Process/Magn_Data_Process1/Mag_Data_Process/Mag_Quality_Estimate ==
  note: TODO: improve this
  mag_normalized_O : Inport
  nominal_inc_deg : Inport  Port=2
  pos_0_valid : Inport  Port=3
  mag_valid : Inport  Port=4
  Mag_Quality : Subsystem
  Multiply : Product  OutDataTypeStr=Inherit: Same as first input
  Switch : Switch  Criteria=u2 > Threshold  SaturateOnIntegerOverflow=off  InputSameDT=off
  default_mag_quality : Constant  Value=0.5  OutDataTypeStr=single
  mag_quality : Outport  VectorParamsAs1DForOutWhenUnconnected=off
  wires:
  pos_0_valid/1 -> Switch/2
  mag_valid/1 -> Multiply/2
  Switch/1 -> Multiply/1
  default_mag_quality/1 -> mag_quality/1, Switch/3
  nominal_inc_deg/1 -> Mag_Quality/1(nominal_inc_deg)
  mag_normalized_O/1 -> Mag_Quality/2(mag_normalized_O)
  Mag_Quality/1(mag_quality) -> Switch/1

== system main_RI_LIEKF_GNSSOutrage/Sensor_Data_Process/Magn_Data_Process1/Mag_Data_Process/WMM_Compensation ==
  WMM_magnitude_uT : Inport
  WMM_declination_deg : Inport  Port=2
  DCM_OB : Inport  Port=3
  mag_B_uT : Inport  Port=4
  pos_0_valid : Inport  Port=5
  Gain : Gain  Gain=-pi/180  OutDataTypeStr=single
  Math Function2 : Math  Operator=transpose  SignedPower=on
  Normlize : Subsystem
  Product{5..8} (4 alike) : Product  Multiplication=Matrix(*)
  Switch3 : Switch  Criteria=u2 > Threshold  SaturateOnIntegerOverflow=off  InputSameDT=off
  psi2DCMz : Subsystem
  safe_divide : Subsystem
      mask Display:
      | port_label('input', 1, 'x', 'texmode', 'on')
      | port_label('input', 2, '÷', 'texmode', 'on')
  mag_normalized_B : Outport  VectorParamsAs1DForOutWhenUnconnected=off
  mag_normalized_O : Outport  Port=2  VectorParamsAs1DForOutWhenUnconnected=off
  wires:
  Gain/1 -> psi2DCMz/1(In1)  "dec_rad"
  WMM_declination_deg/1 -> Gain/1
  mag_B_uT/1 -> Normlize/1(In1), safe_divide/1(u1)  "uT"
  WMM_magnitude_uT/1 -> safe_divide/2(u2)
  safe_divide/1(y) -> Product5/2  "mag_normalized_B"
  DCM_OB/1 -> Product5/1, Math Function2/1, Product7/1
  Product5/1 -> Product6/2  "mag_normalized_O"
  psi2DCMz/1(Out1) -> Product6/1
  Product6/1 -> Switch3/1  "mag_norminal_O"
  Math Function2/1 -> Product8/1  "DCM_BO"
  pos_0_valid/1 -> Switch3/2
  Product8/1 -> mag_normalized_B/1
  Switch3/1 -> mag_normalized_O/1, Product8/2
  Normlize/1(Out1) -> Product7/2
  Product7/1 -> Switch3/3

== system main_RI_LIEKF_GNSSOutrage/Sensor_Data_Process/Magn_Data_Process1/Mag_Data_Process/WMM_LUT ==
  lat_rad : Inport
  lon_rad : Inport  Port=2
  Add : Sum
  Declination_Lookup_Table : LookupNDDirect  Table=wmm_declination  DiagnosticForOutOfRangeInput=Error
  Demux : Demux  Outputs=2
  Inclination_Lookup_Table : LookupNDDirect  Table=wmm_inclination  DiagnosticForOutOfRangeInput=Error
  Magnitude_Lookup_Table : LookupNDDirect  Table=wmm_magnitude  DiagnosticForOutOfRangeInput=Error
  Mux : Mux  Inputs=2
  Saturation1 : Saturate  UpperLimit=size(wmm_magnitude)-1  LowerLimit=0
  offset : Constant  Value=(size(wmm_magnitude)-1)/2  OutDataTypeStr=int32
  rad_to_index : Gain  Gain=180/pi/resolution  OutDataTypeStr=int32
  magnitude_uT : Outport  VectorParamsAs1DForOutWhenUnconnected=off
  declination_deg : Outport  Port=2  VectorParamsAs1DForOutWhenUnconnected=off
  inclination_deg : Outport  Port=3  VectorParamsAs1DForOutWhenUnconnected=off
  wires:
  Inclination_Lookup_Table/1 -> inclination_deg/1
  Declination_Lookup_Table/1 -> declination_deg/1
  Magnitude_Lookup_Table/1 -> magnitude_uT/1
  offset/1 -> Add/2
  Add/1 -> Saturation1/1
  rad_to_index/1 -> Add/1
  lat_rad/1 -> Mux/1
  lon_rad/1 -> Mux/2
  Mux/1 -> rad_to_index/1
  Saturation1/1 -> Demux/1
  Demux/1 -> Magnitude_Lookup_Table/1, Inclination_Lookup_Table/1, Declination_Lookup_Table/1
  Demux/2 -> Inclination_Lookup_Table/2, Magnitude_Lookup_Table/2, Declination_Lookup_Table/2

== system main_RI_LIEKF_GNSSOutrage/Sensor_Data_Process/Magn_Data_Process1/Sensor_Valid/Ever_Valid ==
  in : Inport
  Constant1 : Constant  OutDataTypeStr=uint8
  Delay : Delay  DelayLength=1
  Switch : Switch  Criteria=u2 > Threshold  SaturateOnIntegerOverflow=off  InputSameDT=off
  out : Outport  PortDimensions=1  VectorParamsAs1DForOutWhenUnconnected=off
  wires:
  Constant1/1 -> Switch/1
  Delay/1 -> Switch/3
  in/1 -> Switch/2
  Switch/1 -> out/1, Delay/1

== system main_RI_LIEKF_GNSSOutrage/State estimation/0609bk/Error State Kalman Filter/Cal Phi ==
  Rbn : Inport
  vn : Inport  Port=2
  pn : Inport  Port=3
  Constant : Constant  Value=dt
  MATLAB Function1 : MATLAB Function  TreatAsAtomicUnit=on
  Reshape : Reshape  OutputDimensionality=Column vector (2-D)
  Reshape1 : Reshape  OutputDimensionality=Column vector (2-D)
  Phi : Outport
  wires:
  Reshape1/1 -> MATLAB Function1/2(pn)
  Reshape/1 -> MATLAB Function1/1(vn)
  pn/1 -> Reshape1/1
  vn/1 -> Reshape/1
  Rbn/1 -> MATLAB Function1/3(Rbn)
  MATLAB Function1/1(Phi) -> Phi/1
  Constant/1 -> MATLAB Function1/4(dt)

== system main_RI_LIEKF_GNSSOutrage/State estimation/0609bk/Error State Kalman Filter/Cal Q1 ==
  Constant : Constant  Value=dt  OutDataTypeStr=double
  MATLAB Function1 : MATLAB Function  TreatAsAtomicUnit=on
  Qd : Outport
  wires:
  Constant/1 -> MATLAB Function1/1(dt)
  MATLAB Function1/1(Q) -> Qd/1

== system main_RI_LIEKF_GNSSOutrage/State estimation/0609bk/Error State Kalman Filter/Cal Q2 ==
  Constant : Constant  Value=dt  OutDataTypeStr=double
  MATLAB Function1 : MATLAB Function  TreatAsAtomicUnit=on
  Qd : Outport
  wires:
  MATLAB Function1/1(Q) -> Qd/1
  Constant/1 -> MATLAB Function1/1(dt)

== system main_RI_LIEKF_GNSSOutrage/State estimation/0609bk/Error State Kalman Filter/Extended Kalman Filter1 ==
  Q : Inport
  Enable1 : Inport  Port=2
  y1 : Inport  Port=3
  R1 : Inport  Port=4
  BlockOrdering : Constant  Value=true()  OutDataTypeStr=boolean
  Correct1 : Subsystem  AncestorBlock=sharedTrackingLibrary/Extras/EKFCorrect  TreatAsAtomicUnit=on  SystemSampleTime=p.SampleTimes.MeasurementFcn(1)  mask(EKFCorrect){ProcessedMaskData=p}
      mask init:
      | if strcmp(get_param(bdroot,'SimulationStatus'),'stopped')
      |     pM = [];
      |     SampleTime = [];
      |     DataType = [];
      |     SLFcnsToRegister = {};
      | else
      |     [pM,SampleTime] = ...
      |         matlabshared.tracking.internal.blocks.maskInitializationFcnEKFCorrector...
      |         (gcbh, ProcessedMaskData);
      |     [DataType,SLFcnsToRegister] = ...
      |         matlabshared.tracking.internal.blocks.maskInitializationFcnRegisterSLFcn(ProcessedMaskData, pM);
      | end
      settings: LibrarySourceBlock=sharedTrackingLibrary/Extras/EKFCorrect
  DataStoreMemory - P : DataStoreMemory  DataStoreName=P  InitialValue=p.InitialCovariance  ShowAdditionalParam=off  OutDataTypeStr=p.DataType
  DataStoreMemory - x : DataStoreMemory  DataStoreName=x  InitialValue=p.InitialState  ShowAdditionalParam=off  OutDataTypeStr=p.DataType
  DataTypeConversion_Enable1 : DataTypeConversion  OutDataTypeStr=boolean  SaturateOnIntegerOverflow=off  RndMeth=Floor
  DataTypeConversion_Q : DataTypeConversion  OutDataTypeStr=p.DataType  SaturateOnIntegerOverflow=off  RndMeth=Floor
  DataTypeConversion_R1 : DataTypeConversion  OutDataTypeStr=p.DataType  SaturateOnIntegerOverflow=off  RndMeth=Floor
  DataTypeConversion_uMeas1 : DataTypeConversion  OutDataTypeStr=p.DataType  SaturateOnIntegerOverflow=off  RndMeth=Floor
  DataTypeConversion_uState : DataTypeConversion  OutDataTypeStr=p.DataType  SaturateOnIntegerOverflow=off  RndMeth=Floor
  DataTypeConversion_y1 : DataTypeConversion  OutDataTypeStr=p.DataType  SaturateOnIntegerOverflow=off  RndMeth=Floor
  MeasurementFcn1Inputs : Constant  Value=0  OutDataTypeStr=p.DataType  SampleTime=p.SampleTimes.MeasurementFcn(1)
  Output : Subsystem  TreatAsAtomicUnit=on  SystemSampleTime=p.SampleTimes.Output
  Predict : Subsystem  TreatAsAtomicUnit=on  SystemSampleTime=p.SampleTimes.StateTransitionFcn  mask(EKFPredict){ProcessedMaskData=p}
      mask init:
      | if strcmp(get_param(bdroot,'SimulationStatus'),'stopped')
      |     pS = [];
      |     SampleTime = [];
      |     DataType = [];
      |     SLFcnsToRegister = {};
      | else
      |     [pS,SampleTime] = ...
      |         matlabshared.tracking.internal.blocks.maskInitializationFcnEKFPredictor(ProcessedMaskData);
      |     [DataType,SLFcnsToRegister] = ...
      |         matlabshared.tracking.internal.blocks.maskInitializationFcnRegisterSLFcn(ProcessedMaskData, pS);
      | end
  StateTransitionFcnInputs : Constant  Value=0  OutDataTypeStr=p.DataType  SampleTime=p.SampleTimes.StateTransitionFcn
  checkMeasurementFcn1Signals : S-Function  FunctionName=ekfukfCheckSignals  Parameters=signalCheck.BlockPath, signalCheck.MeasurementFcn{1}.PortNames, signalCheck.MeasurementFcn{1}.SampleTime, signalCheck.DataType, signalCheck.MeasurementFcn{1}.PortDimensions, 1, signalCheck.MeasurementFcn{1}.HasAdditiveNoise  SFunctionDeploymentMode=off  EnableBusSupport=off
  checkStateTransitionFcnSignals : S-Function  FunctionName=ekfukfCheckSignals  Parameters=signalCheck.BlockPath, signalCheck.StateTransitionFcn.PortNames, signalCheck.StateTransitionFcn.SampleTime, signalCheck.DataType, signalCheck.StateTransitionFcn.PortDimensions, 0, signalCheck.StateTransitionFcn.HasAdditiveNoise  SFunctionDeploymentMode=off  EnableBusSupport=off
  xhat : Outport  VectorParamsAs1DForOutWhenUnconnected=off
  P : Outport  Port=2
  wires:
  [AfterOutput] -> Predict/3(uBlockOrdering)
  Output/3(yBlockOrdering) -> [AfterOutput]
  [AfterCorrect] -> Output/1(uBlockOrdering)
  [FirstOperation] -> Correct1/4(uBlockOrdering)
  BlockOrdering/1 -> [FirstOperation]
  DataTypeConversion_uMeas1/1 -> Correct1/3(uMeas)
  DataTypeConversion_R1/1 -> Correct1/2(R)
  MeasurementFcn1Inputs/1 -> DataTypeConversion_uMeas1/1, checkMeasurementFcn1Signals/4
  DataTypeConversion_y1/1 -> Correct1/1(yMeas)
  DataTypeConversion_uState/1 -> Predict/2(uState)
  StateTransitionFcnInputs/1 -> DataTypeConversion_uState/1, checkStateTransitionFcnSignals/2
  Output/1(x) -> xhat/1
  Output/2(P) -> P/1
  DataTypeConversion_Enable1/1 -> Correct1/Enable
  Enable1/1 -> DataTypeConversion_Enable1/1, checkMeasurementFcn1Signals/1
  DataTypeConversion_Q/1 -> Predict/1(Q)
  Q/1 -> DataTypeConversion_Q/1, checkStateTransitionFcnSignals/1
  R1/1 -> DataTypeConversion_R1/1, checkMeasurementFcn1Signals/3
  y1/1 -> DataTypeConversion_y1/1, checkMeasurementFcn1Signals/2
  Correct1/1(yBlockOrdering) -> [AfterCorrect]

== system main_RI_LIEKF_GNSSOutrage/State estimation/0609bk/Error State Kalman Filter/Simulink Function - State Transition ==
  DCM_b_n : Inport
  vn : Inport  Port=2  PortDimensions=[3,1]
  pn : Inport  Port=3  PortDimensions=[3,1]
  Add : Sum
  Cal Phi : Subsystem
  Constant : Constant  Value=dt  OutDataTypeStr=single
  Data Type Conversion1 : DataTypeConversion  OutDataTypeStr=single  SaturateOnIntegerOverflow=off  RndMeth=Floor
  Data Type Conversion6 : DataTypeConversion  OutDataTypeStr=single  SaturateOnIntegerOverflow=off  RndMeth=Floor
  MATLAB Function : MATLAB Function  TreatAsAtomicUnit=on
  Product1 : Product  Multiplication=Matrix(*)
  Product2 : Product  Multiplication=Matrix(*)
  x : ArgIn  DisableCoverage=on  OutDataTypeStr=single  PortDimensions=15  ArgumentName=x
  w : ArgIn  Port=2  OutDataTypeStr=single  PortDimensions=12  ArgumentName=w
  xNext : ArgOut  DisableCoverage=on  OutDataTypeStr=single  PortDimensions=15  ArgumentName=xNext
  wires:
  pn/1 -> Cal Phi/3(pn), MATLAB Function/3(pn)
  vn/1 -> Cal Phi/2(vn), MATLAB Function/2(vn)
  [DCM_b_n] -> Cal Phi/1(Rbn)
  Data Type Conversion6/1 -> Add/2
  Data Type Conversion1/1 -> Add/1
  Cal Phi/1(Phi) -> Product2/1
  DCM_b_n/1 -> [DCM_b_n]
  Constant/1 -> MATLAB Function/4(dt)
  [DCM_b_n] -> MATLAB Function/1(Rbn)
  Add/1 -> xNext/1
  Product1/1 -> Data Type Conversion1/1
  w/1 -> Product1/2
  MATLAB Function/1(G) -> Product1/1
  Product2/1 -> Data Type Conversion6/1
  x/1 -> Product2/2

== system main_RI_LIEKF_GNSSOutrage/State estimation/0609bk/Error State Kalman Filter/Subsystem ==
  data : Inport
  Detect Change : simulink/Logic and Bit Operations/Detect Change  vinit=0  InputProcessing=Columns as channels (frame based)  OutDataTypeStr=boolean
  Selector : Selector  InputPortWidth=3  IndexOptions=Index vector (dialog)  Indices=[3]  OutputSizes=1
  Zero-Order Hold : ZeroOrderHold  SampleTime=0.2
  Zero-Order Hold1 : ZeroOrderHold  SampleTime=0.01
  flag : Outport
  wires:
  Zero-Order Hold1/1 -> Detect Change/1
  Detect Change/1 -> flag/1
  Selector/1 -> Zero-Order Hold1/1
  data/1 -> Zero-Order Hold/1
  Zero-Order Hold/1 -> Selector/1
